simulink model "roach_sync"  (Simulink 7.2)
settings: Solver=ode45  StartTime=0.0  StopTime=16  RelTol=1e-3
libraries: xbsIndex_r4 x70, xps_library x9, casper_library x6
settings Model: Creator=dave  LastModifiedBy=dave
settings OptimizationCC: InitFltsAndDblsToZero=on

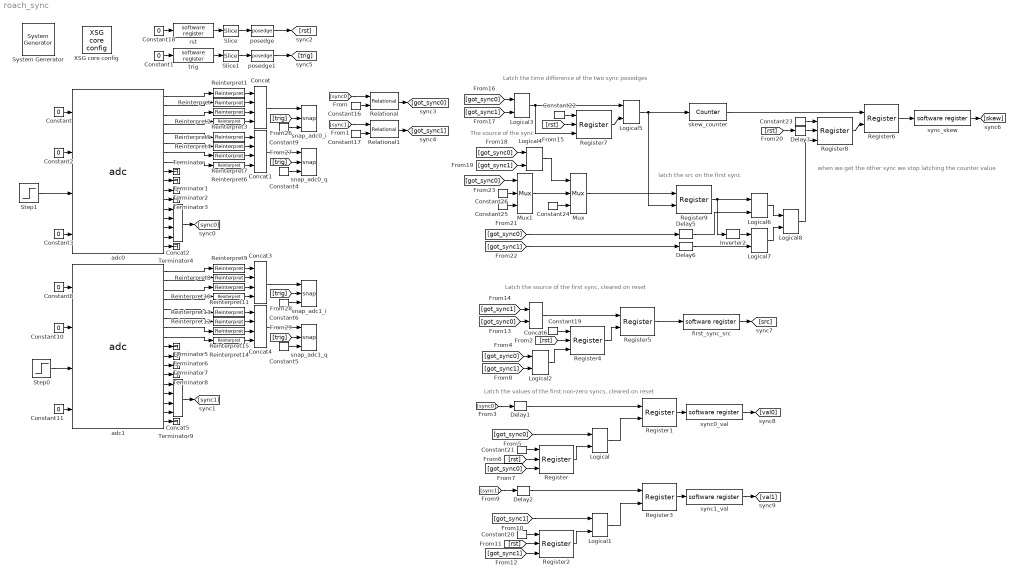
== system roach_sync ==
  note: Latch the values of the first non-zero syncs, cleared on reset
  note: Latch the source of the first sync, cleared on reset
  note: The source of the sync
  note: latch the src on the first sync
  note: when we get the other sync we stop latching the counter value
  note: Latch the time difference of the two sync posedges
  " System Generator" : xbsIndex_r4/ System Generator  Tag=genX  SystemSampleTime=-1  xilinxfamily=virtex5  part=xc5vsx95t  speed=-1  package=ff1136  synthesis_tool=XST  clock_wrapper=Clock Enables  directory=./roach_sync/sysgen  testbench=off  simulink_period=1  sysclk_period=4  dcm_input_clock_period=100  incr_netlist=off  trim_vbits=Everywhere in SubSystem  dbl_ovrd=According to Block Masks  core_generation=According to Block Masks  run_coregen=off  deprecated_control=off  eval_field=0  block_type=sysgen
      settings: block_version=10.1.3
  Concat{,1..5} (6 alike) : xbsIndex_r4/Concat  num_inputs=4  dbl_ovrd=off  block_type=concat
      settings: block_version=10.1.3
  Concat6 : xbsIndex_r4/Concat  num_inputs=2  dbl_ovrd=off  block_type=concat
      settings: block_version=10.1.3
  Constant{,1..3,8,10..11,18} (8 alike) : Constant  Value=0  OutDataType=sfix(16)  OutScaling=2^0
  Constant16 : xbsIndex_r4/Constant  arith_type=Unsigned  const=0  n_bits=4  bin_pt=0  explicit_period=on  period=1  equ=P=C  opselect=C  inp2=PCIN>>17  opr=+  inp1=P  carry=CIN  dbl_ovrd=off  block_type=constant
  Constant17 : xbsIndex_r4/Constant  arith_type=Unsigned  const=0  n_bits=4  bin_pt=0  explicit_period=on  period=1  equ=P=C  opselect=C  inp2=PCIN>>17  opr=+  inp1=P  carry=CIN  dbl_ovrd=off  block_type=constant
  Constant{19..23,25} (6 alike) : xbsIndex_r4/Constant  arith_type=Boolean  const=0  n_bits=1  bin_pt=0  explicit_period=on  period=1  equ=P=C  opselect=C  inp2=PCIN>>17  opr=+  inp1=P  carry=CIN  dbl_ovrd=off  block_type=constant
  Constant24 : xbsIndex_r4/Constant  arith_type=Boolean  const=0  n_bits=2  bin_pt=0  explicit_period=on  period=1  equ=P=C  opselect=C  inp2=PCIN>>17  opr=+  inp1=P  carry=CIN  dbl_ovrd=off  block_type=constant
  Constant26 : xbsIndex_r4/Constant  arith_type=Boolean  const=1  n_bits=1  bin_pt=0  explicit_period=on  period=1  equ=P=C  opselect=C  inp2=PCIN>>17  opr=+  inp1=P  carry=CIN  dbl_ovrd=off  block_type=constant
  Constant{4..6,9} (4 alike) : xbsIndex_r4/Constant  arith_type=Boolean  const=1  n_bits=0  bin_pt=0  explicit_period=on  period=1  equ=P=C  opselect=C  inp2=PCIN>>17  opr=+  inp1=P  carry=CIN  dbl_ovrd=off  block_type=constant
  Delay{1..3,5..6} (5 alike) : xbsIndex_r4/Delay  en=off  latency=1  dbl_ovrd=off  reg_retiming=off  block_type=delay
  Inverter2 : xbsIndex_r4/Inverter  en=off  latency=0  dbl_ovrd=off  block_type=inv
  Logical{,1,4..7} (6 alike) : xbsIndex_r4/Logical  logical_function=AND  inputs=2  en=off  latency=0  precision=Full  arith_type=Unsigned  n_bits=16  bin_pt=0  align_bp=on  dbl_ovrd=off  block_type=logical
  Logical2 : xbsIndex_r4/Logical  logical_function=OR  inputs=2  en=off  latency=0  precision=Full  arith_type=Unsigned  n_bits=16  bin_pt=0  align_bp=on  dbl_ovrd=off  block_type=logical
  Logical3 : xbsIndex_r4/Logical  logical_function=OR  inputs=2  en=off  latency=0  precision=Full  arith_type=Unsigned  n_bits=16  bin_pt=0  align_bp=on  dbl_ovrd=off  block_type=logical
  Logical8 : xbsIndex_r4/Logical  logical_function=OR  inputs=2  en=off  latency=0  precision=Full  arith_type=Unsigned  n_bits=16  bin_pt=0  align_bp=on  dbl_ovrd=off  block_type=logical
  Mux : xbsIndex_r4/Mux  inputs=2  en=off  latency=0  precision=Full  arith_type=Unsigned  n_bits=16  bin_pt=14  quantization=Truncate  overflow=Wrap  dbl_ovrd=off  block_type=mux
  Mux1 : xbsIndex_r4/Mux  inputs=2  en=off  latency=0  precision=Full  arith_type=Unsigned  n_bits=16  bin_pt=14  quantization=Truncate  overflow=Wrap  dbl_ovrd=off  block_type=mux
  Register{,2,4,7..8} (5 alike) : xbsIndex_r4/Register  init=1  rst=on  en=on  dbl_ovrd=off  block_type=register
  Register{1,3,5..6} (4 alike) : xbsIndex_r4/Register  init=1  rst=off  en=on  dbl_ovrd=off  block_type=register
  Register9 : xbsIndex_r4/Register  init=0  rst=off  en=on  dbl_ovrd=off  block_type=register
  Reinterpret{,1..15} (16 alike) : xbsIndex_r4/Reinterpret  force_arith_type=on  arith_type=Unsigned  force_bin_pt=on  bin_pt=0  block_type=reinterpret
      settings: infoedit="Changes signal type without altering the binary representation.   You can changed the signal between signed and unsigned, and relocate the binary point.<P><P>Hardware notes: In hardware this block costs nothing.<P><P>Example:  Suppose the input is 6 bits wide, signed, with 2 fractional bits, and the output is forced to unsigned with 0 fractional bits.  Then an input of -2.0 (1110.00 in binary 2's complement) becomes an output of 56 (111000 in binary)."  block_version=10.1.3
  Relational : xbsIndex_r4/Relational  mode=a!=b  en=off  latency=1  dbl_ovrd=off  block_type=relational
      settings: block_version=10.1.3
  Relational1 : xbsIndex_r4/Relational  mode=a!=b  en=off  latency=1  dbl_ovrd=off  block_type=relational
      settings: block_version=10.1.3
  Slice : xbsIndex_r4/Slice  nbits=1  boolean_output=on  mode=Lower Bit Location + Width  bit1=0  base1=LSB of Input  bit0=0  base0=LSB of Input  dbl_ovrd=off  block_type=slice
      settings: infoedit="Extracts a given range of bits from each input sample and presents it at the output.  The output type is ordinarily unsigned with binary point at zero, but can be Boolean when the slice is one bit wide.<P><P>Hardware notes: In hardware this block costs nothing."  block_version=10.1.3
  Slice1 : xbsIndex_r4/Slice  nbits=1  boolean_output=on  mode=Lower Bit Location + Width  bit1=0  base1=LSB of Input  bit0=0  base0=LSB of Input  dbl_ovrd=off  block_type=slice
      settings: infoedit="Extracts a given range of bits from each input sample and presents it at the output.  The output type is ordinarily unsigned with binary point at zero, but can be Boolean when the slice is one bit wide.<P><P>Hardware notes: In hardware this block costs nothing."  block_version=10.1.3
  Step0 : Step  Time=6  SampleTime=0
  Step1 : Step  Time=5  SampleTime=0
  Terminator{,1..9} (10 alike) : Terminator
  XSG core config : xps_library/XSG core config  Tag=xps:xsg  SystemSampleTime=-1  hw_sys=ROACH:sx95t  ibob_linux=off  clk_src=adc0_clk  iBOB_clk_src=sys_clk  BEE2_ctrl_clk_src=sys_clk  BEE2_usr_clk_src=sys_clk  ROACH_clk_src=adc0_clk  CORR_clk_src=sys_clk  gpio_clk_io_group=iBOB:sma  gpio_clk_bit_index=0  clk_rate=250  sample_period=1  synthesis_tool=XST  mpc_type=powerpc440_ext
  adc0 : xps_library/adc  Tag=xps:adc  SystemSampleTime=-1  adc_brd=adc0  adc_clk_rate=1000  adc_interleave=off  sample_period=1
  adc1 : xps_library/adc  Tag=xps:adc  SystemSampleTime=-1  adc_brd=adc1  adc_clk_rate=1000  adc_interleave=off  sample_period=1
  first_sync_src : xps_library/software register  Tag=xps:sw_reg  SystemSampleTime=-1  io_dir=To Processor  arith_type=Unsigned  bitwidth=32  bin_pt=0  sample_period=1  gw_name=roach_sync_first_sync_src_user_data_in
      link override convert: arith_type=Unsigned  n_bits=32  bin_pt=0
  posedge : casper_library/Misc/posedge  Tag=Rising Edge Detector  SystemSampleTime=-1
  posedge1 : casper_library/Misc/posedge  Tag=Rising Edge Detector  SystemSampleTime=-1
  rst : xps_library/software register  Tag=xps:sw_reg  SystemSampleTime=-1  io_dir=From Processor  arith_type=Unsigned  bitwidth=32  bin_pt=0  sample_period=1  gw_name=roach_sync_rst_user_data_out
      link override roach_sync_rst_user_data_out: arith_type=Unsigned  n_bits=32  bin_pt=0  period=1
  skew_counter : xbsIndex_r4/Counter  cnt_type=Free Running  cnt_to=Inf  operation=Up  start_count=0  cnt_by_val=1  arith_type=Unsigned  n_bits=8  bin_pt=0  load_pin=off  rst=on  en=off  explicit_period=on  period=1  dbl_ovrd=off  use_behavioral_HDL=on  implementation=Fabric  use_rpm=off  block_type=counter
  snap_adc0_i : casper_library/Scopes/snap  SystemSampleTime=-1  nsamples=11
      link override addr/convert: arith_type=Unsigned  n_bits=32  bin_pt=0
      link override bram/convert_din: arith_type=Unsigned
      link override bram/mem/sim_data_in: arith_type=Unsigned
      link override bram/roach_sync_snap_adc0_i_bram_data_out: arith_type=Unsigned
      link override ctrl/roach_sync_snap_adc0_i_ctrl_user_data_out: arith_type=Unsigned  n_bits=32  bin_pt=0  period=1
  snap_adc0_q : casper_library/Scopes/snap  SystemSampleTime=-1  nsamples=11
      link override addr/convert: arith_type=Unsigned  n_bits=32  bin_pt=0
      link override bram/convert_din: arith_type=Unsigned
      link override bram/mem/sim_data_in: arith_type=Unsigned
      link override bram/roach_sync_snap_adc0_q_bram_data_out: arith_type=Unsigned
      link override ctrl/roach_sync_snap_adc0_q_ctrl_user_data_out: arith_type=Unsigned  n_bits=32  bin_pt=0  period=1
  snap_adc1_i : casper_library/Scopes/snap  SystemSampleTime=-1  nsamples=11
      link override addr/convert: arith_type=Unsigned  n_bits=32  bin_pt=0
      link override bram/convert_din: arith_type=Unsigned
      link override bram/mem/sim_data_in: arith_type=Unsigned
      link override bram/roach_sync_snap_adc1_i_bram_data_out: arith_type=Unsigned
      link override ctrl/roach_sync_snap_adc1_i_ctrl_user_data_out: arith_type=Unsigned  n_bits=32  bin_pt=0  period=1
  snap_adc1_q : casper_library/Scopes/snap  SystemSampleTime=-1  nsamples=11
      link override addr/convert: arith_type=Unsigned  n_bits=32  bin_pt=0
      link override bram/convert_din: arith_type=Unsigned
      link override bram/mem/sim_data_in: arith_type=Unsigned
      link override bram/roach_sync_snap_adc1_q_bram_data_out: arith_type=Unsigned
      link override ctrl/roach_sync_snap_adc1_q_ctrl_user_data_out: arith_type=Unsigned  n_bits=32  bin_pt=0  period=1
  sync0_val : xps_library/software register  Tag=xps:sw_reg  SystemSampleTime=-1  io_dir=To Processor  arith_type=Unsigned  bitwidth=32  bin_pt=0  sample_period=1  gw_name=roach_sync_sync0_val_user_data_in
      link override convert: arith_type=Unsigned  n_bits=32  bin_pt=0
  sync1_val : xps_library/software register  Tag=xps:sw_reg  SystemSampleTime=-1  io_dir=To Processor  arith_type=Unsigned  bitwidth=32  bin_pt=0  sample_period=1  gw_name=roach_sync_sync1_val_user_data_in
      link override convert: arith_type=Unsigned  n_bits=32  bin_pt=0
  sync_skew : xps_library/software register  Tag=xps:sw_reg  SystemSampleTime=-1  io_dir=To Processor  arith_type=Unsigned  bitwidth=32  bin_pt=0  sample_period=1  gw_name=roach_sync_sync_skew_user_data_in
      link override convert: arith_type=Unsigned  n_bits=32  bin_pt=0
  trig : xps_library/software register  Tag=xps:sw_reg  SystemSampleTime=-1  io_dir=From Processor  arith_type=Unsigned  bitwidth=32  bin_pt=0  sample_period=1  gw_name=roach_sync_trig_user_data_out
      link override roach_sync_rst_user_data_out: arith_type=Unsigned  n_bits=32  bin_pt=0  period=1
      link override roach_sync_trig_user_data_out: arith_type=Unsigned  n_bits=32  bin_pt=0  period=1
  wires:
  Constant/1 -> adc0/1
  Constant2/1 -> adc0/2
  Constant3/1 -> adc0/4
  Reinterpret1/1 -> Concat/1
  Reinterpret/1 -> Concat/2
  Reinterpret3/1 -> Concat/3
  Reinterpret2/1 -> Concat/4
  adc0/1 -> Reinterpret1/1
  adc0/2 -> Reinterpret/1
  adc0/3 -> Reinterpret3/1
  adc0/4 -> Reinterpret2/1
  Concat/1 -> snap_adc0_i/1
  Reinterpret5/1 -> Concat1/1
  Reinterpret4/1 -> Concat1/2
  Reinterpret7/1 -> Concat1/3
  Reinterpret6/1 -> Concat1/4
  Concat1/1 -> snap_adc0_q/1
  adc0/5 -> Reinterpret5/1
  adc0/6 -> Reinterpret4/1
  adc0/7 -> Reinterpret7/1
  adc0/8 -> Reinterpret6/1
  adc0/9 -> Terminator/1
  adc0/10 -> Terminator1/1
  adc0/11 -> Terminator2/1
  adc0/12 -> Terminator3/1
  adc0/13 -> Concat2/1
  adc0/14 -> Concat2/2
  adc0/15 -> Concat2/3
  adc0/16 -> Concat2/4
  Concat2/1 -> [sync0]
  adc0/17 -> Terminator4/1
  Constant8/1 -> adc1/1
  Step0/1 -> adc1/3
  Constant10/1 -> adc1/2
  Constant11/1 -> adc1/4
  Reinterpret9/1 -> Concat3/1
  Reinterpret8/1 -> Concat3/2
  Reinterpret11/1 -> Concat3/3
  Reinterpret10/1 -> Concat3/4
  adc1/1 -> Reinterpret9/1
  adc1/2 -> Reinterpret8/1
  adc1/3 -> Reinterpret11/1
  adc1/4 -> Reinterpret10/1
  Reinterpret13/1 -> Concat4/1
  Reinterpret12/1 -> Concat4/2
  Reinterpret15/1 -> Concat4/3
  Reinterpret14/1 -> Concat4/4
  adc1/5 -> Reinterpret13/1
  adc1/6 -> Reinterpret12/1
  adc1/7 -> Reinterpret15/1
  adc1/8 -> Reinterpret14/1
  adc1/9 -> Terminator5/1
  adc1/10 -> Terminator6/1
  adc1/11 -> Terminator7/1
  adc1/12 -> Terminator8/1
  adc1/13 -> Concat5/1
  adc1/14 -> Concat5/2
  adc1/15 -> Concat5/3
  adc1/16 -> Concat5/4
  Concat5/1 -> [sync1]
  adc1/17 -> Terminator9/1
  Constant16/1 -> Relational/2
  [sync0] -> Relational/1
  Constant17/1 -> Relational1/2
  [sync1] -> Relational1/1
  Constant18/1 -> rst/1
  rst/1 -> Slice/1
  Slice/1 -> posedge/1
  Constant21/1 -> Register/1
  [rst] -> Register/2
  Relational/1 -> [got_sync0]
  Relational1/1 -> [got_sync1]
  [got_sync0] -> Register/3
  Register/1 -> Logical/2
  [got_sync0] -> Logical/1
  [sync0] -> Delay1/1
  Delay1/1 -> Register1/1
  Register1/1 -> sync0_val/1
  Constant20/1 -> Register2/1
  [rst] -> Register2/2
  [got_sync1] -> Register2/3
  Register2/1 -> Logical1/2
  [got_sync1] -> Logical1/1
  [sync1] -> Delay2/1
  Register3/1 -> sync1_val/1
  Logical/1 -> Register1/2
  Delay2/1 -> Register3/1
  Logical1/1 -> Register3/2
  [rst] -> Register4/2
  Constant19/1 -> Register4/1
  [got_sync0] -> Logical2/1
  [got_sync1] -> Logical2/2
  Logical2/1 -> Register4/3
  [got_sync1] -> Concat6/1
  [got_sync0] -> Concat6/2
  Concat6/1 -> Register5/1
  Register4/1 -> Register5/2
  Register5/1 -> first_sync_src/1
  Register6/1 -> sync_skew/1
  [rst] -> Register7/2
  Constant22/1 -> Register7/1
  [got_sync0] -> Logical3/1
  [got_sync1] -> Logical3/2
  [got_sync0] -> Logical4/1
  [got_sync1] -> Logical4/2
  Logical3/1 -> Logical5/1, Register7/3
  Logical5/1 -> skew_counter/1, Register9/2
  skew_counter/1 -> Register6/1
  [rst] -> Delay3/1
  Constant23/1 -> Register8/1
  Register8/1 -> Register6/2
  [got_sync0] -> Delay5/1
  [got_sync1] -> Delay6/1
  Logical4/1 -> Mux/1
  Constant24/1 -> Mux/3
  Mux1/1 -> Mux/2
  [got_sync0] -> Mux1/1
  Constant26/1 -> Mux1/2
  Constant25/1 -> Mux1/3
  Mux/1 -> Register9/1
  Delay3/1 -> Register8/2
  Register9/1 -> Inverter2/1, Logical6/1
  Delay5/1 -> Logical6/2
  Delay6/1 -> Logical7/2
  Logical6/1 -> Logical8/1
  Logical7/1 -> Logical8/2
  Logical8/1 -> Register8/3
  sync_skew/1 -> [skew]
  Step1/1 -> adc0/3
  Constant1/1 -> trig/1
  trig/1 -> Slice1/1
  Slice1/1 -> posedge1/1
  posedge/1 -> [rst]
  posedge1/1 -> [trig]
  [trig] -> snap_adc0_i/2
  Constant9/1 -> snap_adc0_i/3
  [trig] -> snap_adc0_q/2
  Constant4/1 -> snap_adc0_q/3
  Concat3/1 -> snap_adc1_i/1
  Concat4/1 -> snap_adc1_q/1
  [trig] -> snap_adc1_i/2
  Constant6/1 -> snap_adc1_i/3
  [trig] -> snap_adc1_q/2
  Constant5/1 -> snap_adc1_q/3
  sync0_val/1 -> [val0]
  sync1_val/1 -> [val1]
  first_sync_src/1 -> [src]
  Register7/1 -> Logical5/2
  Inverter2/1 -> Logical7/1
